simulink model "simbarra_step"  (R2018a)
settings: Solver=VariableStepAuto  StartTime=0.0  StopTime=10.0  RelTol=1e-3
values from neighbouring files (symbols this model uses):
  Ts = mean(diff(ts))    [controller.m]    (also in identify.m; identify_v2.m; simubarra1.m = 0.01)
undefined symbols (not defined in the file or in its folder): Atrue, Btrue, Ctrue, Dtrue
settings Model: Creator=mange  LastModifiedBy=mange

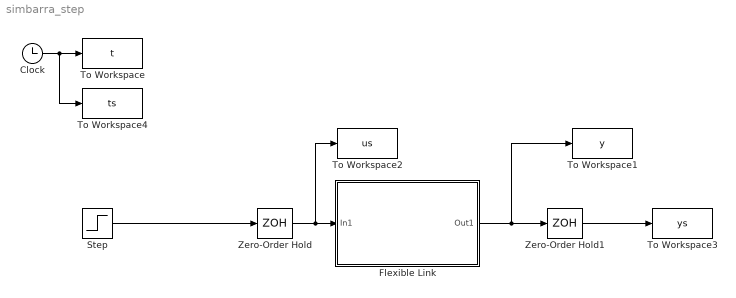
== system simbarra_step ==
  Clock : Clock
  Flexible Link : Subsystem
      mask Display: image('quanserlink.jpg')
  Step : Step  SampleTime=Ts
  To Workspace : ToWorkspace  VariableName=t  SampleTime=-1
  To Workspace1 : ToWorkspace  VariableName=y  SampleTime=-1
  To Workspace2 : ToWorkspace  VariableName=us  SampleTime=Ts
  To Workspace3 : ToWorkspace  VariableName=ys  SampleTime=Ts
  To Workspace4 : ToWorkspace  VariableName=ts  SampleTime=Ts
  Zero-Order Hold : ZeroOrderHold  SampleTime=Ts
  Zero-Order Hold1 : ZeroOrderHold  SampleTime=Ts
  wires:
  Zero-Order Hold1/1 -> To Workspace3/1
  Flexible Link/1(Out1) -> Zero-Order Hold1/1, To Workspace1/1
  Zero-Order Hold/1 -> Flexible Link/1(In1), To Workspace2/1
  Clock/1 -> To Workspace/1, To Workspace4/1
  Step/1 -> Zero-Order Hold/1

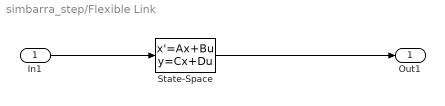
== system simbarra_step/Flexible Link ==
  In1 : Inport
  State-Space : StateSpace  A=Atrue  B=Btrue  C=Ctrue  D=Dtrue  InitialCondition=0
  Out1 : Outport
  wires:
  In1/1 -> State-Space/1
  State-Space/1 -> Out1/1
